simulink model "motor_controller"  (R2020b)
settings: Solver=VariableStepAuto  StartTime=0.0  StopTime=0.2  RelTol=1e-3
model workspace (MAT data in the model file):
  Kd = Simulink.Parameter
  Kd.Value = 120
  Kd.DataType = 'auto'
  Kd.Dimensions = [1 1]
  Ki = Simulink.Parameter
  Ki.Value = 200
  Ki.DataType = 'auto'
  Ki.Dimensions = [1 1]
  Kp = Simulink.Parameter
  Kp.Value = 350
  Kp.DataType = 'auto'
  Kp.Dimensions = [1 1]
settings Model: Creator=gokul  LastModifiedBy=gokul
settings DataIOCC: SaveOutput=off  SaveTime=off

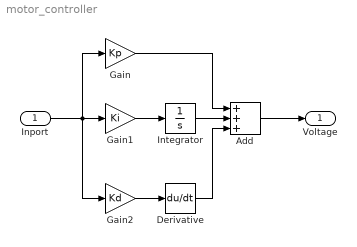
== system motor_controller ==
  Inport : Inport  OutDataTypeStr=double  PortDimensions=1  SampleTime=0
  Add : Sum  Inputs=+++
  Derivative : Derivative
  Gain : Gain  Gain=Kp
  Gain1 : Gain  Gain=Ki
  Gain2 : Gain  Gain=Kd
  Integrator : Integrator
  Voltage : Outport  OutDataTypeStr=double  PortDimensions=1  SampleTime=0
  wires:
  Add/1 -> Voltage/1
  Gain2/1 -> Derivative/1
  Derivative/1 -> Add/3
  Inport/1 -> Gain1/1, Gain/1, Gain2/1
  Integrator/1 -> Add/2
  Gain/1 -> Add/1
  Gain1/1 -> Integrator/1
